simulink model "HQEV_MiL_20160830_integrate_r2017a"  (Simulink 8.9)
settings: Solver=FixedStepDiscrete  StartTime=0.0  StopTime=inf  FixedStep=0.01  RelTol=1e-3  EnableMultiTasking=on
PostLoadFcn:
  | , if any(exist('dsrtsu_mdlpostloadfcn', 'file') == [2, 3, 6]), try dsrtsu_mdlpostloadfcn('Execute', bdroot); catch fprintf('Error in PostLoadFcn (dsrtsu_mdlpostloadfcn) for model "%s":\n %s\n', bdroot, lasterr); end, end,
values from neighbouring files (symbols this model uses):
  Bat_C_Ah = 36    [parameter_V1.mat]
  Bat_ocv_xIndex = [5 10 20 30 40 50 60 70 80 90 95]    [parameter_V1.mat]
  Bat_ocv_z = [329 332 340 345 347 351 358 372 377 386 391]    [parameter_V1.mat]
  Bat_R_ohm_z = [4.41 3.46 1.57 1.07 0.76 0.63 0.55 0.44 0.41 0.4 0.4 3.14 ... (66 elements, 11x6)]    [parameter_V1.mat]
  Bat_SOC_Init = 90    [parameter_V1.mat]
  Env_hum_pct_Ambient = 30    [parameter_V1.mat]
  Env_Slope_deg = 0    [parameter_V1.mat]
  Env_Temp_degC_Ambient = 25    [parameter_V1.mat]
  Env_v_kmph_HWind = 0    [parameter_V1.mat]
  Reducer_F_i = 7.23    [parameter_V1.mat]
  Reducer_R_i = 7.23    [parameter_V1.mat]
  Veh =     [parameter_V1.mat]
  Veh_A_m2_Fr = 2.246    [parameter_V1.mat]
  Veh_F_Brake =     [parameter_V1.mat]
  Veh_fac_AirDrag = 0.326    [parameter_V1.mat]
  Veh_fac_WhDragFrict_0 = 0.011    [parameter_V1.mat]
  Veh_g_mps2_C = 9.81    [parameter_V1.mat]
  Veh_GainBrake =     [parameter_V1.mat]
  Veh_h_m_COGHigh = 0.5    [parameter_V1.mat]
  Veh_J_kgm2_Wh = 1.3635    [parameter_V1.mat]
  Veh_L_m_AxlBas = 2.63    [parameter_V1.mat]
  Veh_M_kg = 1427    [parameter_V1.mat]
  Veh_mu_Brake = 0.4    [parameter_V1.mat]
  Veh_mu_Tyre =     [parameter_V1.mat]
  Veh_num_FrictPair = 8    [parameter_V1.mat]
  Veh_pct_Brk = 70    [parameter_V1.mat]
  Veh_r_dyn =     [parameter_V1.mat]
  Veh_r_m_BrkDisk = 0.136    [parameter_V1.mat]
  Veh_rho_kgpm3_Air = 1.2258    [parameter_V1.mat]
undefined symbols (not defined in the file or in its folder): DiscIntNeverNeededParam, p_bool_False_M, p_bool_True_M
libraries: BaseOperationLib_Browser x38, simulink x8, DTQC_lib x1, ERR_lib x1, MQM_lib x1, PTCL_lib x1, PUD_lib x1, TQD_lib x1, TQR_lib x1, VMM_lib x1, ACCA_lib x1, BBCA_lib x1
(part 15 of 15)

== system HQEV_MiL_20160830_integrate_r2017a/MiL/Test_Integration/MCU_RR/MCU/MCU/Subsystem14/Torque_Control/Subsystem/Max_Torque/Max_Gen_Torque_Subsystem ==
  EM_Volt : Inport
  EM_spd : Inport  Port=2
  Bus Creator : BusCreator  Inputs=3
  Constant : Constant  Value=-1
  Constant1 : Constant  Value=-1
  Constant2 : Constant  Value=-1
  Interpolation_2nd : Subsystem
  Max_Gen_Torque_at_300V : Lookup  InputValues=|  Table=|  LookUpMeth=Interpolation-Use End Values
      InputValues=|
      | [0
      | 500
      | 1000
      | 1500
      | 2000
      | 2500
      | 2700
      | 3000
      | 3500
      | 4000
      | 4500
      | 5000
      | 5500
      | 6000
      | 6500
      | 7000
      | 7500
      | 8000
      | 8500
      | 9000
      | 9500
      | 10000
      | 10500
      | 11000
      | 11500
      | 12000
      | ]
      Table=|
      | [340
      | 340
      | 340
      | 340
      | 340
      | 340
      | 340
      | 316
      | 272
      | 236
      | 206
      | 180
      | 160
      | 144
      | 130
      | 120
      | 110
      | 102
      | 94
      | 88
      | 84
      | 78
      | 74
      | 70
      | 66
      | 64
      | ]
  Max_Gen_Torque_at_340V : Lookup  InputValues=|  Table=|  LookUpMeth=Interpolation-Use End Values
      InputValues=|
      | [0
      | 500
      | 1000
      | 1500
      | 2000
      | 2500
      | 3000
      | 3100
      | 3500
      | 4000
      | 4500
      | 5000
      | 5500
      | 6000
      | 6500
      | 7000
      | 7500
      | 8000
      | 8500
      | 9000
      | 9500
      | 10000
      | 10500
      | 11000
      | 11500
      | 12000
      | ]
      Table=|
      | [340
      | 340
      | 340
      | 340
      | 340
      | 340
      | 340
      | 340
      | 310
      | 272
      | 240
      | 212
      | 190
      | 170
      | 154
      | 140
      | 128
      | 118
      | 110
      | 104
      | 96
      | 90
      | 86
      | 82
      | 78
      | 74
      | ]
  Max_Mot_Torque_at_280V : Lookup  InputValues=|  Table=|  LookUpMeth=Interpolation-Use End Values
      InputValues=|
      | [0
      | 500
      | 1000
      | 1500
      | 2000
      | 2500
      | 3000
      | 3500
      | 4000
      | 4500
      | 5000
      | 5500
      | 6000
      | 6500
      | 7000
      | 7500
      | 8000
      | 8500
      | 9000
      | 9500
      | 10000
      | 10500
      | 11000
      | 11500
      | 12000
      | ]
      Table=|
      | [340
      | 340
      | 340
      | 340
      | 340
      | 340
      | 296
      | 252
      | 218
      | 188
      | 166
      | 146
      | 132
      | 120
      | 110
      | 102
      | 94
      | 88
      | 82
      | 76
      | 72
      | 68
      | 64
      | 62
      | 58
      | ]
  Product : Product  RndMeth=Zero
  Product1 : Product  RndMeth=Zero
  Product2 : Product  RndMeth=Zero
  abs_val : Subsystem
  Out1 : Outport
  wires:
  Interpolation_2nd/1(Out1) -> Out1/1
  EM_spd/1 -> abs_val/1(In1)
  Bus Creator/1 -> Interpolation_2nd/2(In2)
  EM_Volt/1 -> Interpolation_2nd/1(In1)
  abs_val/1(Out1) -> Max_Gen_Torque_at_340V/1, Max_Gen_Torque_at_300V/1, Max_Mot_Torque_at_280V/1
  Max_Mot_Torque_at_280V/1 -> Product/1
  Max_Gen_Torque_at_300V/1 -> Product1/1
  Max_Gen_Torque_at_340V/1 -> Product2/1
  Constant/1 -> Product/2
  Constant1/1 -> Product1/2
  Constant2/1 -> Product2/2
  Product/1 -> Bus Creator/1  "at280V"
  Product1/1 -> Bus Creator/2  "at300V"
  Product2/1 -> Bus Creator/3  "at340V"

== system HQEV_MiL_20160830_integrate_r2017a/MiL/Test_Integration/MCU_RR/MCU/MCU/Subsystem14/Torque_Control/Subsystem/Max_Torque/Max_Mot_Torque_Subsystem ==
  EM_Volt : Inport
  EM_spd : Inport  Port=2
  Bus Creator : BusCreator  Inputs=3
  Interpolation_2nd : Subsystem
  Max_Gen_Torque_at_300V : Lookup  InputValues=|  Table=|  LookUpMeth=Interpolation-Use End Values
      InputValues=|
      | [0
      | 500
      | 1000
      | 1500
      | 2000
      | 2500
      | 2700
      | 3000
      | 3500
      | 4000
      | 4500
      | 5000
      | 5500
      | 6000
      | 6500
      | 7000
      | 7500
      | 8000
      | 8500
      | 9000
      | 9500
      | 10000
      | 10500
      | 11000
      | 11500
      | 12000
      | ]
      Table=|
      | [340
      | 340
      | 340
      | 340
      | 340
      | 340
      | 340
      | 316
      | 272
      | 236
      | 206
      | 180
      | 160
      | 144
      | 130
      | 120
      | 110
      | 102
      | 94
      | 88
      | 84
      | 78
      | 74
      | 70
      | 66
      | 64
      | ]
  Max_Gen_Torque_at_340V : Lookup  InputValues=|  Table=|  LookUpMeth=Interpolation-Use End Values
      InputValues=|
      | [0
      | 500
      | 1000
      | 1500
      | 2000
      | 2500
      | 3000
      | 3100
      | 3500
      | 4000
      | 4500
      | 5000
      | 5500
      | 6000
      | 6500
      | 7000
      | 7500
      | 8000
      | 8500
      | 9000
      | 9500
      | 10000
      | 10500
      | 11000
      | 11500
      | 12000
      | ]
      Table=|
      | [340
      | 340
      | 340
      | 340
      | 340
      | 340
      | 340
      | 340
      | 310
      | 272
      | 240
      | 212
      | 190
      | 170
      | 154
      | 140
      | 128
      | 118
      | 110
      | 104
      | 96
      | 90
      | 86
      | 82
      | 78
      | 74
      | ]
  Max_Mot_Torque_at_280V : Lookup  InputValues=|  Table=|  LookUpMeth=Interpolation-Use End Values
      InputValues=|
      | [0
      | 500
      | 1000
      | 1500
      | 2000
      | 2500
      | 3000
      | 3500
      | 4000
      | 4500
      | 5000
      | 5500
      | 6000
      | 6500
      | 7000
      | 7500
      | 8000
      | 8500
      | 9000
      | 9500
      | 10000
      | 10500
      | 11000
      | 11500
      | 12000
      | ]
      Table=|
      | [340
      | 340
      | 340
      | 340
      | 340
      | 340
      | 296
      | 252
      | 218
      | 188
      | 166
      | 146
      | 132
      | 120
      | 110
      | 102
      | 94
      | 88
      | 82
      | 76
      | 72
      | 68
      | 64
      | 62
      | 58
      | ]
  abs_val : Subsystem
  Out1 : Outport
  wires:
  abs_val/1(Out1) -> Max_Mot_Torque_at_280V/1, Max_Gen_Torque_at_300V/1, Max_Gen_Torque_at_340V/1
  Max_Mot_Torque_at_280V/1 -> Bus Creator/1  "at280V"
  Max_Gen_Torque_at_300V/1 -> Bus Creator/2  "at300V"
  Max_Gen_Torque_at_340V/1 -> Bus Creator/3  "at340V"
  EM_Volt/1 -> Interpolation_2nd/1(In1)
  Bus Creator/1 -> Interpolation_2nd/2(In2)
  EM_spd/1 -> abs_val/1(In1)
  Interpolation_2nd/1(Out1) -> Out1/1

== system HQEV_MiL_20160830_integrate_r2017a/MiL/Test_Integration/MCU_FF/MCU/MCU/Torque_Control/Subsystem/Max_Torque/Max_Gen_Torque_Subsystem/Interpolation_2nd/0V_280V ==
  In1 : Inport
  Bus Selector : BusSelector  OutputSignals=at280V
  Out1 : Outport
  wires:
  Bus Selector/1 -> Out1/1  "<at280V>"
  In1/1 -> Bus Selector/1

== system HQEV_MiL_20160830_integrate_r2017a/MiL/Test_Integration/MCU_FF/MCU/MCU/Torque_Control/Subsystem/Max_Torque/Max_Gen_Torque_Subsystem/Interpolation_2nd/280V_300V ==
  In1 : Inport
  In2 : Inport  Port=2
  Add : Sum
  Bus Selector : BusSelector  OutputSignals=at280V
  Bus Selector1 : BusSelector  OutputSignals=at300V
  Constant : Constant  Value=280
  Constant1 : Constant  Value=300
  Constant2 : Constant  Value=20
  Constant3 : Constant  Value=20
  Divide : Product  Inputs=*/
  Divide1 : Product  Inputs=*/
  Product : Product  RndMeth=Zero
  Product1 : Product  RndMeth=Zero
  Subtract : Sum  Inputs=+-
  Subtract1 : Sum  Inputs=+-
  Out1 : Outport
  wires:
  Add/1 -> Out1/1
  Product1/1 -> Add/2
  Product/1 -> Add/1
  Bus Selector/1 -> Product1/2  "<at280V>"
  Bus Selector1/1 -> Product/2  "<at300V>"
  In2/1 -> Bus Selector1/1, Bus Selector/1
  Divide1/1 -> Product1/1
  Divide/1 -> Product/1
  Constant3/1 -> Divide/2
  Constant2/1 -> Divide1/2
  Subtract/1 -> Divide1/1
  Subtract1/1 -> Divide/1
  Constant1/1 -> Subtract1/1
  Constant/1 -> Subtract/2
  In1/1 -> Subtract1/2, Subtract/1

== system HQEV_MiL_20160830_integrate_r2017a/MiL/Test_Integration/MCU_FF/MCU/MCU/Torque_Control/Subsystem/Max_Torque/Max_Gen_Torque_Subsystem/Interpolation_2nd/300V_340V ==
  In1 : Inport
  In2 : Inport  Port=2
  Add : Sum
  Bus Selector : BusSelector  OutputSignals=at300V
  Bus Selector1 : BusSelector  OutputSignals=at340V
  Constant : Constant  Value=300
  Constant1 : Constant  Value=340
  Constant2 : Constant  Value=40
  Constant3 : Constant  Value=40
  Divide : Product  Inputs=*/
  Divide1 : Product  Inputs=*/
  Product : Product  RndMeth=Zero
  Product1 : Product  RndMeth=Zero
  Subtract : Sum  Inputs=+-
  Subtract1 : Sum  Inputs=+-
  Out1 : Outport
  wires:
  In1/1 -> Subtract/1, Subtract1/2
  Constant/1 -> Subtract/2
  Constant1/1 -> Subtract1/1
  Subtract1/1 -> Divide/1
  Subtract/1 -> Divide1/1
  Constant2/1 -> Divide1/2
  Constant3/1 -> Divide/2
  Divide/1 -> Product/1
  Divide1/1 -> Product1/1
  In2/1 -> Bus Selector/1, Bus Selector1/1
  Bus Selector1/1 -> Product/2  "<at340V>"
  Bus Selector/1 -> Product1/2  "<at300V>"
  Product/1 -> Add/1
  Product1/1 -> Add/2
  Add/1 -> Out1/1

== system HQEV_MiL_20160830_integrate_r2017a/MiL/Test_Integration/MCU_FF/MCU/MCU/Torque_Control/Subsystem/Max_Torque/Max_Gen_Torque_Subsystem/Interpolation_2nd/340V_inf ==
  In1 : Inport
  Bus Selector : BusSelector  OutputSignals=at340V
  Out1 : Outport
  wires:
  Bus Selector/1 -> Out1/1  "<at340V>"
  In1/1 -> Bus Selector/1

== system HQEV_MiL_20160830_integrate_r2017a/MiL/Test_Integration/MCU_FF/MCU/MCU/Torque_Control/Subsystem/Max_Torque/Max_Gen_Torque_Subsystem/Interpolation_2nd/MM ==
  In1 : Inport
  Lookup Table : Lookup  InputValues=[0 280 281 300 301 340 341 500]  Table=[1 1 2 2 3 3 4 4]
  Out1 : Outport
  wires:
  In1/1 -> Lookup Table/1
  Lookup Table/1 -> Out1/1

== system HQEV_MiL_20160830_integrate_r2017a/MiL/Test_Integration/MCU_FF/MCU/MCU/Torque_Control/Subsystem/Max_Torque/Max_Mot_Torque_Subsystem/Interpolation_2nd/0V_280V ==
  In1 : Inport
  Bus Selector : BusSelector  OutputSignals=at280V
  Out1 : Outport
  wires:
  In1/1 -> Bus Selector/1
  Bus Selector/1 -> Out1/1  "<at280V>"

== system HQEV_MiL_20160830_integrate_r2017a/MiL/Test_Integration/MCU_FF/MCU/MCU/Torque_Control/Subsystem/Max_Torque/Max_Mot_Torque_Subsystem/Interpolation_2nd/280V_300V ==
  In1 : Inport
  In2 : Inport  Port=2
  Add : Sum
  Bus Selector : BusSelector  OutputSignals=at280V
  Bus Selector1 : BusSelector  OutputSignals=at300V
  Constant : Constant  Value=280
  Constant1 : Constant  Value=300
  Constant2 : Constant  Value=20
  Constant3 : Constant  Value=20
  Divide : Product  Inputs=*/
  Divide1 : Product  Inputs=*/
  Product : Product  RndMeth=Zero
  Product1 : Product  RndMeth=Zero
  Subtract : Sum  Inputs=+-
  Subtract1 : Sum  Inputs=+-
  Out1 : Outport
  wires:
  In1/1 -> Subtract/1, Subtract1/2
  Constant/1 -> Subtract/2
  Constant1/1 -> Subtract1/1
  Subtract1/1 -> Divide/1
  Subtract/1 -> Divide1/1
  Constant2/1 -> Divide1/2
  Constant3/1 -> Divide/2
  Divide/1 -> Product/1
  Divide1/1 -> Product1/1
  In2/1 -> Bus Selector/1, Bus Selector1/1
  Bus Selector1/1 -> Product/2  "<at300V>"
  Bus Selector/1 -> Product1/2  "<at280V>"
  Product/1 -> Add/1
  Product1/1 -> Add/2
  Add/1 -> Out1/1

== system HQEV_MiL_20160830_integrate_r2017a/MiL/Test_Integration/MCU_FF/MCU/MCU/Torque_Control/Subsystem/Max_Torque/Max_Mot_Torque_Subsystem/Interpolation_2nd/300V_340V ==
  In1 : Inport
  In2 : Inport  Port=2
  Add : Sum
  Bus Selector : BusSelector  OutputSignals=at300V
  Bus Selector1 : BusSelector  OutputSignals=at340V
  Constant : Constant  Value=300
  Constant1 : Constant  Value=340
  Constant2 : Constant  Value=40
  Constant3 : Constant  Value=40
  Divide : Product  Inputs=*/
  Divide1 : Product  Inputs=*/
  Product : Product  RndMeth=Zero
  Product1 : Product  RndMeth=Zero
  Subtract : Sum  Inputs=+-
  Subtract1 : Sum  Inputs=+-
  Out1 : Outport
  wires:
  Add/1 -> Out1/1
  Product1/1 -> Add/2
  Product/1 -> Add/1
  Bus Selector/1 -> Product1/2  "<at300V>"
  Bus Selector1/1 -> Product/2  "<at340V>"
  In2/1 -> Bus Selector1/1, Bus Selector/1
  Divide1/1 -> Product1/1
  Divide/1 -> Product/1
  Constant3/1 -> Divide/2
  Constant2/1 -> Divide1/2
  Subtract/1 -> Divide1/1
  Subtract1/1 -> Divide/1
  Constant1/1 -> Subtract1/1
  Constant/1 -> Subtract/2
  In1/1 -> Subtract1/2, Subtract/1

== system HQEV_MiL_20160830_integrate_r2017a/MiL/Test_Integration/MCU_FF/MCU/MCU/Torque_Control/Subsystem/Max_Torque/Max_Mot_Torque_Subsystem/Interpolation_2nd/340V_inf ==
  In1 : Inport
  Bus Selector : BusSelector  OutputSignals=at340V
  Out1 : Outport
  wires:
  In1/1 -> Bus Selector/1
  Bus Selector/1 -> Out1/1  "<at340V>"

== system HQEV_MiL_20160830_integrate_r2017a/MiL/Test_Integration/MCU_FF/MCU/MCU/Torque_Control/Subsystem/Max_Torque/Max_Mot_Torque_Subsystem/Interpolation_2nd/MM ==
  In1 : Inport
  Lookup Table : Lookup  InputValues=[0 280 281 300 301 340 341 500]  Table=[1 1 2 2 3 3 4 4]
  Out1 : Outport
  wires:
  Lookup Table/1 -> Out1/1
  In1/1 -> Lookup Table/1

== system HQEV_MiL_20160830_integrate_r2017a/MiL/Test_Integration/MCU_RR/MCU/MCU/Subsystem14/Torque_Control/Subsystem/Max_Torque/Max_Gen_Torque_Subsystem/Interpolation_2nd ==
  In1 : Inport
  In2 : Inport  Port=2
  0V_280V : Subsystem
  280V_300V : Subsystem
  300V_340V : Subsystem
  340V_inf : Subsystem
  MM : Subsystem
  Multiport Switch : MultiPortSwitch  Inputs=4
  Out1 : Outport
  wires:
  In2/1 -> 300V_340V/2(In2), 340V_inf/1(In1), 280V_300V/2(In2), 0V_280V/1(In1)
  Multiport Switch/1 -> Out1/1
  MM/1(Out1) -> Multiport Switch/1
  In1/1 -> 300V_340V/1(In1), 280V_300V/1(In1), MM/1(In1)
  340V_inf/1(Out1) -> Multiport Switch/5
  300V_340V/1(Out1) -> Multiport Switch/4
  280V_300V/1(Out1) -> Multiport Switch/3
  0V_280V/1(Out1) -> Multiport Switch/2

== system HQEV_MiL_20160830_integrate_r2017a/MiL/Test_Integration/MCU_RR/MCU/MCU/Subsystem14/Torque_Control/Subsystem/Max_Torque/Max_Gen_Torque_Subsystem/abs_val ==
  In1 : Inport
  Constant : Constant  Value=0
  Constant1 : Constant  Value=-1
  Product : Product  RndMeth=Zero
  Relational Operator : RelationalOperator  OutDataTypeStr=boolean  RndMeth=Nearest
  Switch : Switch  Criteria=u2 ~= 0
  Out1 : Outport
  wires:
  Switch/1 -> Out1/1
  In1/1 -> Product/1, Relational Operator/1, Switch/1
  Constant1/1 -> Product/2
  Product/1 -> Switch/3
  Relational Operator/1 -> Switch/2
  Constant/1 -> Relational Operator/2

== system HQEV_MiL_20160830_integrate_r2017a/MiL/Test_Integration/MCU_RR/MCU/MCU/Subsystem14/Torque_Control/Subsystem/Max_Torque/Max_Mot_Torque_Subsystem/Interpolation_2nd ==
  In1 : Inport
  In2 : Inport  Port=2
  0V_280V : Subsystem
  280V_300V : Subsystem
  300V_340V : Subsystem
  340V_inf : Subsystem
  MM : Subsystem
  Multiport Switch : MultiPortSwitch  Inputs=4
  Out1 : Outport
  wires:
  0V_280V/1(Out1) -> Multiport Switch/2
  280V_300V/1(Out1) -> Multiport Switch/3
  300V_340V/1(Out1) -> Multiport Switch/4
  340V_inf/1(Out1) -> Multiport Switch/5
  In1/1 -> MM/1(In1), 280V_300V/1(In1), 300V_340V/1(In1)
  MM/1(Out1) -> Multiport Switch/1
  Multiport Switch/1 -> Out1/1
  In2/1 -> 0V_280V/1(In1), 280V_300V/2(In2), 340V_inf/1(In1), 300V_340V/2(In2)

== system HQEV_MiL_20160830_integrate_r2017a/MiL/Test_Integration/MCU_RR/MCU/MCU/Subsystem14/Torque_Control/Subsystem/Max_Torque/Max_Mot_Torque_Subsystem/abs_val ==
  In1 : Inport
  Constant : Constant  Value=0
  Constant1 : Constant  Value=-1
  Product : Product  RndMeth=Zero
  Relational Operator : RelationalOperator  OutDataTypeStr=boolean  RndMeth=Nearest
  Switch : Switch  Criteria=u2 ~= 0
  Out1 : Outport
  wires:
  Constant/1 -> Relational Operator/2
  Relational Operator/1 -> Switch/2
  Product/1 -> Switch/3
  Constant1/1 -> Product/2
  In1/1 -> Switch/1, Relational Operator/1, Product/1
  Switch/1 -> Out1/1

== system HQEV_MiL_20160830_integrate_r2017a/MiL/Test_Integration/MCU_RR/MCU/MCU/Subsystem14/Torque_Control/Subsystem/Max_Torque/Max_Gen_Torque_Subsystem/Interpolation_2nd/0V_280V ==
  In1 : Inport
  Bus Selector : BusSelector  OutputSignals=at280V
  Out1 : Outport
  wires:
  Bus Selector/1 -> Out1/1  "<at280V>"
  In1/1 -> Bus Selector/1

== system HQEV_MiL_20160830_integrate_r2017a/MiL/Test_Integration/MCU_RR/MCU/MCU/Subsystem14/Torque_Control/Subsystem/Max_Torque/Max_Gen_Torque_Subsystem/Interpolation_2nd/280V_300V ==
  In1 : Inport
  In2 : Inport  Port=2
  Add : Sum
  Bus Selector : BusSelector  OutputSignals=at280V
  Bus Selector1 : BusSelector  OutputSignals=at300V
  Constant : Constant  Value=280
  Constant1 : Constant  Value=300
  Constant2 : Constant  Value=20
  Constant3 : Constant  Value=20
  Divide : Product  Inputs=*/
  Divide1 : Product  Inputs=*/
  Product : Product  RndMeth=Zero
  Product1 : Product  RndMeth=Zero
  Subtract : Sum  Inputs=+-
  Subtract1 : Sum  Inputs=+-
  Out1 : Outport
  wires:
  Add/1 -> Out1/1
  Product1/1 -> Add/2
  Product/1 -> Add/1
  Bus Selector/1 -> Product1/2  "<at280V>"
  Bus Selector1/1 -> Product/2  "<at300V>"
  In2/1 -> Bus Selector1/1, Bus Selector/1
  Divide1/1 -> Product1/1
  Divide/1 -> Product/1
  Constant3/1 -> Divide/2
  Constant2/1 -> Divide1/2
  Subtract/1 -> Divide1/1
  Subtract1/1 -> Divide/1
  Constant1/1 -> Subtract1/1
  Constant/1 -> Subtract/2
  In1/1 -> Subtract1/2, Subtract/1

== system HQEV_MiL_20160830_integrate_r2017a/MiL/Test_Integration/MCU_RR/MCU/MCU/Subsystem14/Torque_Control/Subsystem/Max_Torque/Max_Gen_Torque_Subsystem/Interpolation_2nd/300V_340V ==
  In1 : Inport
  In2 : Inport  Port=2
  Add : Sum
  Bus Selector : BusSelector  OutputSignals=at300V
  Bus Selector1 : BusSelector  OutputSignals=at340V
  Constant : Constant  Value=300
  Constant1 : Constant  Value=340
  Constant2 : Constant  Value=40
  Constant3 : Constant  Value=40
  Divide : Product  Inputs=*/
  Divide1 : Product  Inputs=*/
  Product : Product  RndMeth=Zero
  Product1 : Product  RndMeth=Zero
  Subtract : Sum  Inputs=+-
  Subtract1 : Sum  Inputs=+-
  Out1 : Outport
  wires:
  In1/1 -> Subtract/1, Subtract1/2
  Constant/1 -> Subtract/2
  Constant1/1 -> Subtract1/1
  Subtract1/1 -> Divide/1
  Subtract/1 -> Divide1/1
  Constant2/1 -> Divide1/2
  Constant3/1 -> Divide/2
  Divide/1 -> Product/1
  Divide1/1 -> Product1/1
  In2/1 -> Bus Selector/1, Bus Selector1/1
  Bus Selector1/1 -> Product/2  "<at340V>"
  Bus Selector/1 -> Product1/2  "<at300V>"
  Product/1 -> Add/1
  Product1/1 -> Add/2
  Add/1 -> Out1/1

== system HQEV_MiL_20160830_integrate_r2017a/MiL/Test_Integration/MCU_RR/MCU/MCU/Subsystem14/Torque_Control/Subsystem/Max_Torque/Max_Gen_Torque_Subsystem/Interpolation_2nd/340V_inf ==
  In1 : Inport
  Bus Selector : BusSelector  OutputSignals=at340V
  Out1 : Outport
  wires:
  Bus Selector/1 -> Out1/1  "<at340V>"
  In1/1 -> Bus Selector/1

== system HQEV_MiL_20160830_integrate_r2017a/MiL/Test_Integration/MCU_RR/MCU/MCU/Subsystem14/Torque_Control/Subsystem/Max_Torque/Max_Gen_Torque_Subsystem/Interpolation_2nd/MM ==
  In1 : Inport
  Lookup Table : Lookup  InputValues=[0 280 281 300 301 340 341 500]  Table=[1 1 2 2 3 3 4 4]
  Out1 : Outport
  wires:
  In1/1 -> Lookup Table/1
  Lookup Table/1 -> Out1/1

== system HQEV_MiL_20160830_integrate_r2017a/MiL/Test_Integration/MCU_RR/MCU/MCU/Subsystem14/Torque_Control/Subsystem/Max_Torque/Max_Mot_Torque_Subsystem/Interpolation_2nd/0V_280V ==
  In1 : Inport
  Bus Selector : BusSelector  OutputSignals=at280V
  Out1 : Outport
  wires:
  In1/1 -> Bus Selector/1
  Bus Selector/1 -> Out1/1  "<at280V>"

== system HQEV_MiL_20160830_integrate_r2017a/MiL/Test_Integration/MCU_RR/MCU/MCU/Subsystem14/Torque_Control/Subsystem/Max_Torque/Max_Mot_Torque_Subsystem/Interpolation_2nd/280V_300V ==
  In1 : Inport
  In2 : Inport  Port=2
  Add : Sum
  Bus Selector : BusSelector  OutputSignals=at280V
  Bus Selector1 : BusSelector  OutputSignals=at300V
  Constant : Constant  Value=280
  Constant1 : Constant  Value=300
  Constant2 : Constant  Value=20
  Constant3 : Constant  Value=20
  Divide : Product  Inputs=*/
  Divide1 : Product  Inputs=*/
  Product : Product  RndMeth=Zero
  Product1 : Product  RndMeth=Zero
  Subtract : Sum  Inputs=+-
  Subtract1 : Sum  Inputs=+-
  Out1 : Outport
  wires:
  In1/1 -> Subtract/1, Subtract1/2
  Constant/1 -> Subtract/2
  Constant1/1 -> Subtract1/1
  Subtract1/1 -> Divide/1
  Subtract/1 -> Divide1/1
  Constant2/1 -> Divide1/2
  Constant3/1 -> Divide/2
  Divide/1 -> Product/1
  Divide1/1 -> Product1/1
  In2/1 -> Bus Selector/1, Bus Selector1/1
  Bus Selector1/1 -> Product/2  "<at300V>"
  Bus Selector/1 -> Product1/2  "<at280V>"
  Product/1 -> Add/1
  Product1/1 -> Add/2
  Add/1 -> Out1/1

== system HQEV_MiL_20160830_integrate_r2017a/MiL/Test_Integration/MCU_RR/MCU/MCU/Subsystem14/Torque_Control/Subsystem/Max_Torque/Max_Mot_Torque_Subsystem/Interpolation_2nd/300V_340V ==
  In1 : Inport
  In2 : Inport  Port=2
  Add : Sum
  Bus Selector : BusSelector  OutputSignals=at300V
  Bus Selector1 : BusSelector  OutputSignals=at340V
  Constant : Constant  Value=300
  Constant1 : Constant  Value=340
  Constant2 : Constant  Value=40
  Constant3 : Constant  Value=40
  Divide : Product  Inputs=*/
  Divide1 : Product  Inputs=*/
  Product : Product  RndMeth=Zero
  Product1 : Product  RndMeth=Zero
  Subtract : Sum  Inputs=+-
  Subtract1 : Sum  Inputs=+-
  Out1 : Outport
  wires:
  Add/1 -> Out1/1
  Product1/1 -> Add/2
  Product/1 -> Add/1
  Bus Selector/1 -> Product1/2  "<at300V>"
  Bus Selector1/1 -> Product/2  "<at340V>"
  In2/1 -> Bus Selector1/1, Bus Selector/1
  Divide1/1 -> Product1/1
  Divide/1 -> Product/1
  Constant3/1 -> Divide/2
  Constant2/1 -> Divide1/2
  Subtract/1 -> Divide1/1
  Subtract1/1 -> Divide/1
  Constant1/1 -> Subtract1/1
  Constant/1 -> Subtract/2
  In1/1 -> Subtract1/2, Subtract/1

== system HQEV_MiL_20160830_integrate_r2017a/MiL/Test_Integration/MCU_RR/MCU/MCU/Subsystem14/Torque_Control/Subsystem/Max_Torque/Max_Mot_Torque_Subsystem/Interpolation_2nd/340V_inf ==
  In1 : Inport
  Bus Selector : BusSelector  OutputSignals=at340V
  Out1 : Outport
  wires:
  In1/1 -> Bus Selector/1
  Bus Selector/1 -> Out1/1  "<at340V>"

== system HQEV_MiL_20160830_integrate_r2017a/MiL/Test_Integration/MCU_RR/MCU/MCU/Subsystem14/Torque_Control/Subsystem/Max_Torque/Max_Mot_Torque_Subsystem/Interpolation_2nd/MM ==
  In1 : Inport
  Lookup Table : Lookup  InputValues=[0 280 281 300 301 340 341 500]  Table=[1 1 2 2 3 3 4 4]
  Out1 : Outport
  wires:
  Lookup Table/1 -> Out1/1
  In1/1 -> Lookup Table/1

== stateflow chart MiL/Test_Integration/Charger/Charger/Charger/Charger/Chart ==
  state Idle
    en:State=1;
    (default) -> (junction 7)
    (junction 7) -> (junction 8) : {
        | Do_Idle;
        | }
  state Work
    en:State=2;
    (default) -> (junction 11)
    (junction 11) -> (junction 12) : {
        | Do_Work;
        | }
  state Fault
    en:State=4;
    (default) -> (junction 15)
    (junction 15) -> (junction 16) : {
        | Do_Fault
        | }
  state Abnormal
    en:State=3;
    (default) -> (junction 19)
    (junction 19) -> (junction 20) : {
        | Do_Abnormal;
        | }
  Idle -> Fault [order 3] : [Charger_Fault]
  Fault -> Idle : [Charger_Fault==0]
  (default) -> Idle
  Idle -> Work [order 1] : [Charge_Enable]
  Work -> Fault [order 1] : [Charger_Fault]
  Work -> Idle [order 2] : [Charge_Finish]
  Work -> Abnormal [order 3] : [Charger_Abnormal]
  Idle -> Abnormal [order 2] : [Charger_Abnormal]
  Abnormal -> Fault [order 2] : [Charger_Fault]
  Abnormal -> Idle [order 1] : [Charger_Abnormal==0]
  data: Charger_Fault input double; Charge_Enable input double; Charge_Finish input double; Charger_Abnormal input double; State output double
  events: Do_Idle output FUNCTION_CALL_EVENT; Do_Work output FUNCTION_CALL_EVENT; Do_Abnormal output FUNCTION_CALL_EVENT; Do_Fault output FUNCTION_CALL_EVENT

== stateflow chart MiL/Test_Integration/Charger/Charger/Charger/Charger/Idle/Subsystem/Chart ==
  state No_Connect
    du:RechargeRequest=0;
  state CC_Connect
    state WakeUp
      du:RechargeRequest=1;
    state AC_220V
      du:RechargeRequest=0;
    state AC_0V
      du:RechargeRequest=0;
      ex:counter=0;
    (default) -> AC_220V
    (junction 49) -> AC_220V [order 1] : [counter>10]
    (junction 49) -> WakeUp [order 2]
    AC_220V -> AC_0V : [PowerOff]
    WakeUp -> (junction 49) : {counter++;}
    AC_0V -> WakeUp : [PowerOn]
  No_Connect -> CC_Connect : [CC>0]
  (default) -> No_Connect
  CC_Connect -> No_Connect : [CC==0]
  data: RechargeRequest output double; PowerOn input double; PowerOff input double; CC input double; counter local double

== stateflow chart MiL/Test_Integration/MCU_FF/MCU/MCU/Chart ==
  state GSD
    en:MCU1_TMStatus=5;
    (default) -> (junction 75)
    GSD -> (junction 75)
    (junction 75) -> (junction 76) : {GSD_Act;
        | }
  state Invalid
    en:MCU1_TMStatus=7;
    (default) -> (junction 80)
    Invalid -> (junction 80)
    (junction 80) -> (junction 81) : {Invalid_Act;
        | }
  state Sleep
    en:MCU1_TMStatus=0;
    (default) -> (junction 85)
    Sleep -> (junction 85) [order 1]
    (junction 85) -> (junction 86) : {
        | Sleep_Act;
        | }
  state Init
    en:MCU1_TMStatus=0;
    (default) -> (junction 90)
    Init -> (junction 90) [order 1]
    (junction 90) -> (junction 91) : {
        | Init_Act;
        | }
  state Torque_Control
    en:MCU1_TMStatus=3;
    (default) -> (junction 95)
    Torque_Control -> (junction 95) [order 1]
    (junction 95) -> (junction 96) : {Torque_Control_Act;
        | }
  state Precharge
    en:MCU1_TMStatus=1;
    (default) -> (junction 100)
    Precharge -> (junction 100) [order 1]
    (junction 100) -> (junction 101) : {Precharge_Act;
        | }
  state Standby
    en:MCU1_TMStatus=2;
    (default) -> (junction 105)
    Standby -> (junction 105) [order 1]
    (junction 105) -> (junction 106) : {
        | Standby_Act;
        | }
  state Stop
    en:MCU1_TMStatus=4;
    (default) -> (junction 110)
    Stop -> (junction 110) [order 1]
    (junction 110) -> (junction 111) : {Stop_Act;
        | }
  state Rapid_Discharge
    en:MCU1_TMStatus=6;
    (default) -> (junction 115)
    Rapid_Discharge -> (junction 115) [order 1]
    (junction 115) -> (junction 116) : {Rapid_Discharge_Act;
        | }
  (default) -> Sleep
  Torque_Control -> GSD [order 3] : [1==0]
  Rapid_Discharge -> Sleep [order 2] : [SleepInd==1&&Uc1<10]
  Sleep -> Init [order 1] : [SleepInd==0]
  Torque_Control -> Invalid [order 4] : [1==0]
  Rapid_Discharge -> Init [order 1] : [SleepInd==0]
  Init -> Precharge [order 1]
  Standby -> Torque_Control [order 2] : [HCU_StatusTMRequestToMCU1==1 ...
      | &&HCU_StopRequestToMCU1==0]
  Torque_Control -> Standby [order 2] : [HCU_StatusTMRequestToMCU1==0 ...
      | &&HCU_StopRequestToMCU1==0]
  Torque_Control -> Stop [order 1] : [HCU_StopRequestToMCU1==1]
  Precharge -> Standby [order 1] : [BMS_MainPlusContactorState==1 ...
      | &&BMS_MainMinusContactorCoilState==1 ...
      | ||Charger_OutputVoltage >= 360]
  Standby -> Stop [order 1] : [HCU_StopRequestToMCU1==1]
  Stop -> Rapid_Discharge [order 1] : [BMS_MainPlusContactorState==0 ...
      | &&BMS_PrechargeContactorCoilState==0 ...
      | &&HCU_RapidDischargeCmdToMCU1==1]
  data: MCU1_TMStatus output double; SleepInd input double; BMS_MainPlusContactorState input double; BMS_MainMinusContactorCoilState input double; HCU_StatusTMRequestToMCU1 input double; HCU_StopRequestToMCU1 input double; BMS_PrechargeContactorCoilState input double; HCU_RapidDischargeCmdToMCU1 input double; Uc1 input double; Charger_OutputVoltage input double
  events: Sleep_Act output FUNCTION_CALL_EVENT; Init_Act output FUNCTION_CALL_EVENT; Precharge_Act output FUNCTION_CALL_EVENT; Standby_Act output FUNCTION_CALL_EVENT; Torque_Control_Act output FUNCTION_CALL_EVENT; Stop_Act output FUNCTION_CALL_EVENT; GSD_Act output FUNCTION_CALL_EVENT; Rapid_Discharge_Act output FUNCTION_CALL_EVENT; Invalid_Act output FUNCTION_CALL_EVENT

== stateflow chart MiL/Test_Integration/MCU_RR/MCU/MCU/Subsystem14/Chart ==
  state GSD
    en:MCU1_TMStatus=5;
    (default) -> (junction 163)
    GSD -> (junction 163)
    (junction 163) -> (junction 164) : {GSD_Act;
        | }
  state Invalid
    en:MCU1_TMStatus=7;
    (default) -> (junction 168)
    Invalid -> (junction 168)
    (junction 168) -> (junction 169) : {Invalid_Act;
        | }
  state Sleep
    en:MCU1_TMStatus=0;
    (default) -> (junction 173)
    Sleep -> (junction 173) [order 1]
    (junction 173) -> (junction 174) : {
        | Sleep_Act;
        | }
  state Init
    en:MCU1_TMStatus=0;
    (default) -> (junction 178)
    Init -> (junction 178) [order 1]
    (junction 178) -> (junction 179) : {
        | Init_Act;
        | }
  state Torque_Control
    en:MCU1_TMStatus=3;
    (default) -> (junction 183)
    Torque_Control -> (junction 183) [order 1]
    (junction 183) -> (junction 184) : {Torque_Control_Act;
        | }
  state Precharge
    en:MCU1_TMStatus=1;
    (default) -> (junction 188)
    Precharge -> (junction 188) [order 1]
    (junction 188) -> (junction 189) : {Precharge_Act;
        | }
  state Standby
    en:MCU1_TMStatus=2;
    (default) -> (junction 193)
    Standby -> (junction 193) [order 1]
    (junction 193) -> (junction 194) : {
        | Standby_Act;
        | }
  state Stop
    en:MCU1_TMStatus=4;
    (default) -> (junction 198)
    Stop -> (junction 198) [order 1]
    (junction 198) -> (junction 199) : {Stop_Act;
        | }
  state Rapid_Discharge
    en:MCU1_TMStatus=6;
    (default) -> (junction 203)
    Rapid_Discharge -> (junction 203) [order 1]
    (junction 203) -> (junction 204) : {Rapid_Discharge_Act;
        | }
  (default) -> Sleep
  Torque_Control -> GSD [order 3] : [1==0]
  Rapid_Discharge -> Sleep [order 2] : [SleepInd==1&&Uc1<10]
  Sleep -> Init [order 1] : [SleepInd==0]
  Torque_Control -> Invalid [order 4] : [1==0]
  Rapid_Discharge -> Init [order 1] : [SleepInd==0]
  Init -> Precharge [order 1]
  Standby -> Torque_Control [order 2] : [HCU_StatusTMRequestToMCU1==1 ...
      | &&HCU_StopRequestToMCU1==0]
  Torque_Control -> Standby [order 2] : [HCU_StatusTMRequestToMCU1==0 ...
      | &&HCU_StopRequestToMCU1==0]
  Torque_Control -> Stop [order 1] : [HCU_StopRequestToMCU1==1]
  Precharge -> Standby [order 1] : [BMS_MainPlusContactorState==1 ...
      | &&BMS_MainMinusContactorCoilState==1 ...
      | ||Charger_OutputVoltage >= 360]
  Standby -> Stop [order 1] : [HCU_StopRequestToMCU1==1]
  Stop -> Rapid_Discharge [order 1] : [BMS_MainPlusContactorState==0 ...
      | &&BMS_PrechargeContactorCoilState==0 ...
      | &&HCU_RapidDischargeCmdToMCU1==1]
  data: MCU1_TMStatus output double; SleepInd input double; BMS_MainPlusContactorState input double; BMS_MainMinusContactorCoilState input double; HCU_StatusTMRequestToMCU1 input double; HCU_StopRequestToMCU1 input double; BMS_PrechargeContactorCoilState input double; HCU_RapidDischargeCmdToMCU1 input double; Uc1 input double; Charger_OutputVoltage input double
  events: Sleep_Act output FUNCTION_CALL_EVENT; Init_Act output FUNCTION_CALL_EVENT; Precharge_Act output FUNCTION_CALL_EVENT; Standby_Act output FUNCTION_CALL_EVENT; Torque_Control_Act output FUNCTION_CALL_EVENT; Stop_Act output FUNCTION_CALL_EVENT; GSD_Act output FUNCTION_CALL_EVENT; Rapid_Discharge_Act output FUNCTION_CALL_EVENT; Invalid_Act output FUNCTION_CALL_EVENT

== stateflow chart MiL/Test_Integration/Epark/Subsystem/Epark/Epark_Process/EPark_Process ==
  state Parked
    en:
    cnt=0;
    st_ParkLoceState=2;
    bool_ParkSensor=1;
    bool_DriveSensor=0;
  state Unparking
    en:
    cnt=0;
    st_ParkLoceState=4;
    bool_ParkSensor=1;
    bool_DriveSensor=0;
    du:
    cnt++;
  state Unparked
    en:
    cnt=0;
    st_ParkLoceState=5;
    bool_ParkSensor=0;
    bool_DriveSensor=1;
  state Parking
    en:
    cnt=0;
    st_ParkLoceState=1;
    bool_ParkSensor=0;
    bool_DriveSensor=0;
    du:
    cnt++;
  (default) -> Parked
  Parking -> Parked : [cnt>100]
  Parked -> Unparking : [st_EparkRequestIn==st_pUnparkRequest_M]
  Unparked -> Parking : [st_EparkRequestIn==st_pParkRequest_M]
  Unparking -> Unparked : [cnt>100]
  data: st_EparkRequestIn input double; st_pParkRequest_M input double; st_pUnparkRequest_M input double; st_ParkLoceState output double; bool_ParkSensor output double; bool_DriveSensor output double; cnt local double
